simulink model "convertidor_simu"  (R2025a)
settings: Solver=VariableStepAuto  StartTime=0.0  StopTime=0.10  RelTol=1e-3
PreLoadFcn:
  | L = 2;
  | R=10 ;
  | C=10;
  | Vin = 32;
settings Model: Creator=Chris  LastModifiedBy=Chris

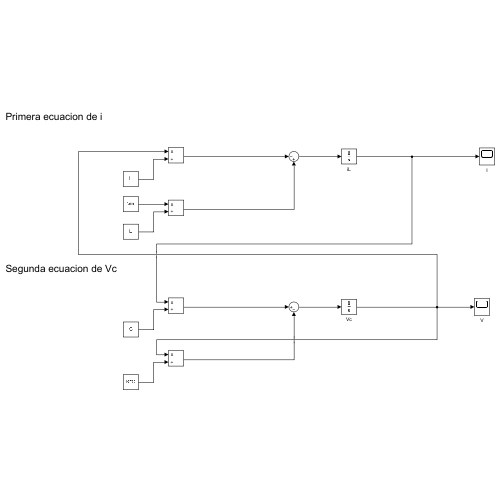
[thumbnail: Simulink's stored preview of the top-level diagram]
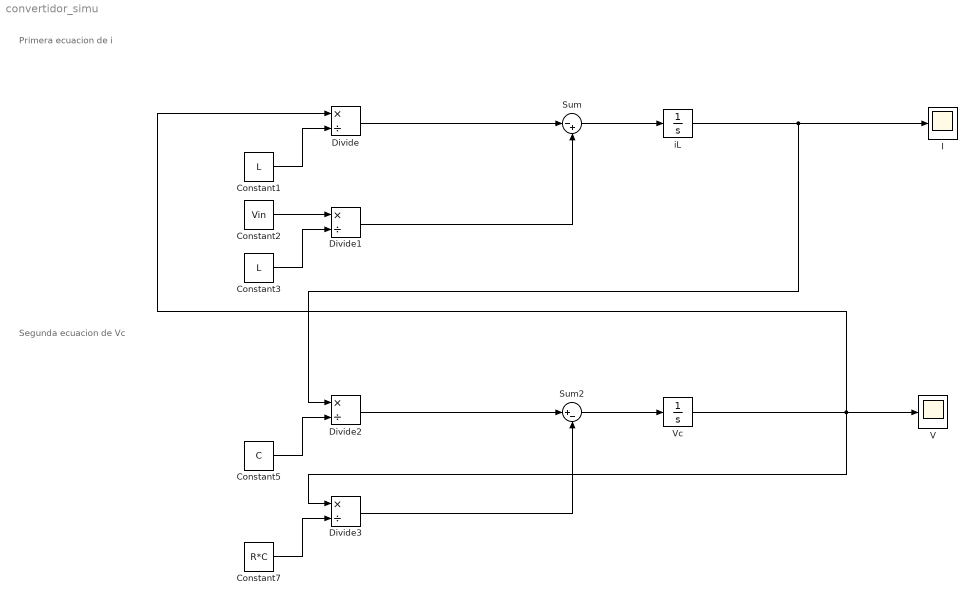
== system convertidor_simu ==
  note: Primera ecuacion de i
  note: Segunda ecuacion de Vc
  Constant1 : Constant  Value=L
  Constant2 : Constant  Value=Vin
  Constant3 : Constant  Value=L
  Constant5 : Constant  Value=C
  Constant7 : Constant  Value=R*C
  Divide{,1..3} (4 alike) : Product  Inputs=*/
  I : Scope
      settings: ActiveDisplayYMinimum=-0.1547474816043255  ActiveDisplayYMaximum=1.5727837821096535
  Sum : Sum  Inputs=|-+
  Sum2 : Sum  Inputs=|+-
  V : Scope
      settings: ActiveDisplayYMinimum=-0.0009996251006733094  ActiveDisplayYMaximum=0.0089966259060597874
  Vc : Integrator
  iL : Integrator
  wires:
  Divide/1 -> Sum/1
  Vc/1 -> Divide3/1, V/1, Divide/1
  Constant1/1 -> Divide/2
  Constant3/1 -> Divide1/2
  Constant2/1 -> Divide1/1
  Divide1/1 -> Sum/2
  Divide3/1 -> Sum2/2
  Constant5/1 -> Divide2/2
  Constant7/1 -> Divide3/2
  iL/1 -> Divide2/1, I/1
  Divide2/1 -> Sum2/1
  Sum/1 -> iL/1
  Sum2/1 -> Vc/1
